simulink model "Three_blade_H_VAWT_Model"  (R2018b)
settings: Solver=FixedStepAuto  StartTime=0.0  StopTime=10  FixedStep=0.01  RelTol=1e-3
values from neighbouring files (symbols this model uses):
  A0 = 0    [Three_blade_H_VAWT_init.m]    (also in Three_blade_H_VAWT_pre_post.m)
  a1 = 0.01    [Three_blade_H_VAWT_init.m]    (also in Three_blade_H_VAWT_pre_post.m)
  a11 = 0.8    [Three_blade_H_VAWT_init.m]    (also in Three_blade_H_VAWT_pre_post.m)
  a12 = 0.2    [Three_blade_H_VAWT_init.m]    (also in Three_blade_H_VAWT_pre_post.m)
  a2 = 0.08    [Three_blade_H_VAWT_init.m]    (also in Three_blade_H_VAWT_pre_post.m)
  a21 = 0.5    [Three_blade_H_VAWT_init.m]    (also in Three_blade_H_VAWT_pre_post.m)
  a22 = 0.5    [Three_blade_H_VAWT_init.m]    (also in Three_blade_H_VAWT_pre_post.m)
  A_wind = 10    [Three_blade_H_VAWT_init.m]    (also in Three_blade_H_VAWT_pre_post.m)
  ACD1 = 12    [Three_blade_H_VAWT_init.m]    (also in Three_blade_H_VAWT_pre_post.m)
  ACL1 = 15    [Three_blade_H_VAWT_init.m]    (also in Three_blade_H_VAWT_pre_post.m)
  AR = Blade_Length/Chord    (= 10)    [Three_blade_H_VAWT_init.m]    (also in Three_blade_H_VAWT_pre_post.m = 40)
  blade1_pitch = 0    [Three_blade_H_VAWT_pre_post.m]
  blade1_radius = 20    [Three_blade_H_VAWT_pre_post.m]
  blade2_pitch = 0    [Three_blade_H_VAWT_pre_post.m]
  blade2_radius = 20    [Three_blade_H_VAWT_pre_post.m]
  blade3_pitch = 0    [Three_blade_H_VAWT_pre_post.m]
  blade3_radius = 20    [Three_blade_H_VAWT_pre_post.m]
  Blade_Length = 40    [Three_blade_H_VAWT_init.m]    (also in Three_blade_H_VAWT_pre_post.m)
  C_l_NACA0012_spline = spline(angles, C_l_NACA0012, [0:1:360])    [Three_blade_H_VAWT_init.m]    (also in Three_blade_H_VAWT_pre_post.m)
  CD0 = 0.005    [Three_blade_H_VAWT_init.m]    (also in Three_blade_H_VAWT_pre_post.m)
  CD1_max = 0.017    [Three_blade_H_VAWT_init.m]    (also in Three_blade_H_VAWT_pre_post.m)
  CD2_max = 1.8    [Three_blade_H_VAWT_init.m]    (also in Three_blade_H_VAWT_pre_post.m)
  CL1_max = 1.4    [Three_blade_H_VAWT_init.m]    (also in Three_blade_H_VAWT_pre_post.m)
  CL2_max = 1.2    [Three_blade_H_VAWT_init.m]    (also in Three_blade_H_VAWT_pre_post.m)
  D = 10^6    (= 1000000)    [Three_blade_H_VAWT_init.m]    (also in Three_blade_H_VAWT_pre_post.m)
  eta_g = 0.9    [Three_blade_H_VAWT_init.m]    (also in Three_blade_H_VAWT_pre_post.m)
  h1 = 1    [Three_blade_H_VAWT_init.m]    (also in Three_blade_H_VAWT_pre_post.m)
  h2 = 1    [Three_blade_H_VAWT_init.m]    (also in Three_blade_H_VAWT_pre_post.m)
  Jg = 15.8    [Three_blade_H_VAWT_init.m]    (also in Three_blade_H_VAWT_pre_post.m)
  K = 6*10^7    (= 60000000)    [Three_blade_H_VAWT_init.m]    (also in Three_blade_H_VAWT_pre_post.m)
  N = 100    [Three_blade_H_VAWT_init.m]    (also in Three_blade_H_VAWT_pre_post.m)
  phi11 = 0    [Three_blade_H_VAWT_init.m]    (also in Three_blade_H_VAWT_pre_post.m)
  phi12 = pi/2    (= 1.57079632679)    [Three_blade_H_VAWT_init.m]    (also in Three_blade_H_VAWT_pre_post.m)
  phi21 = 0    [Three_blade_H_VAWT_init.m]    (also in Three_blade_H_VAWT_pre_post.m)
  phi22 = pi/2    (= 1.57079632679)    [Three_blade_H_VAWT_init.m]    (also in Three_blade_H_VAWT_pre_post.m)
  Planform_A = Blade_Length*Chord    (= 160)    [Three_blade_H_VAWT_init.m]    (also in Three_blade_H_VAWT_pre_post.m = 40)
  rho = 1.225    [Three_blade_H_VAWT_init.m]    (also in Three_blade_H_VAWT_pre_post.m; sim_init_junior_project.m)
  S1 = 0.6/6    (= 0.1)    [Three_blade_H_VAWT_init.m]    (also in Three_blade_H_VAWT_pre_post.m)
  v_gustmax = v_wind    (= 5)    [Three_blade_H_VAWT_init.m]    (also in Three_blade_H_VAWT_pre_post.m)
  v_wind = 5    [Three_blade_H_VAWT_init.m]    (also in Three_blade_H_VAWT_pre_post.m)
  w_gust = (2*pi)/(30)    (= 0.209439510239)    [Three_blade_H_VAWT_init.m]    (also in Three_blade_H_VAWT_pre_post.m)
  w_wind = (2*pi)*5    (= 31.4159265359)    [Three_blade_H_VAWT_init.m]    (also in Three_blade_H_VAWT_pre_post.m)
  wind_vector_i = [50,0,0]    [Three_blade_H_VAWT_pre_post.m]
undefined symbols (not defined in the file or in its folder): Bg, C_Tg, C_Tr, c_wg, c_wr, Cg, Cr, J_g, Kg, Kr, L, magnitude, R2, Re, tau_e
libraries: vrlib x6, dspmathops x6
(part 1 of 2)
settings Model: Creator=Ryan  LastModifiedBy=Ryan
settings DataIOCC: InspectSignalLogs=on
settings SFSimCC: SimUseLocalCustomCode=off
settings RTWCC: RTWUseLocalCustomCode=off
settings CodeAppCC: StateflowObjectComments=on

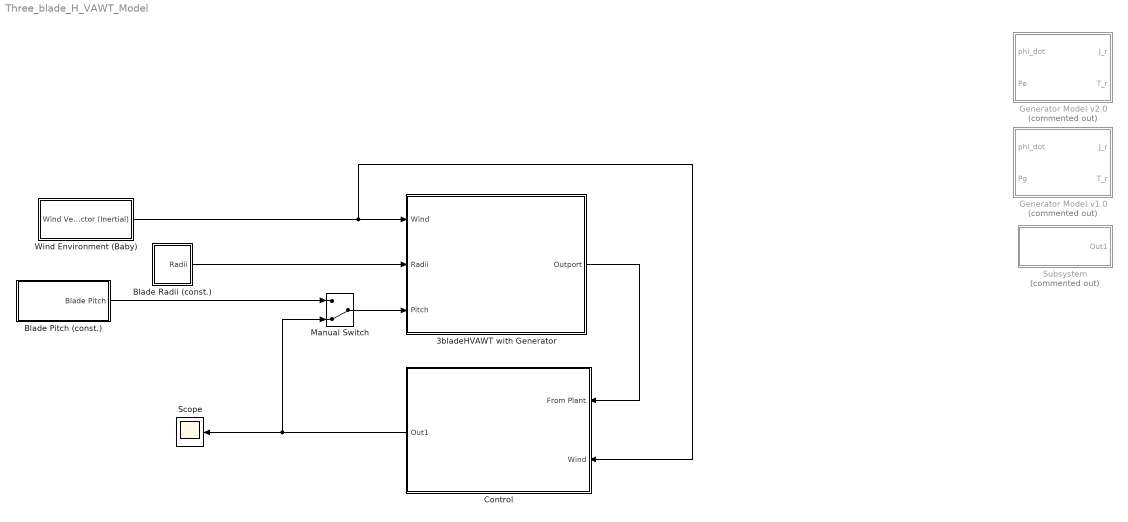
== system Three_blade_H_VAWT_Model ==
  3bladeHVAWT with Generator : Subsystem
  Blade Pitch (const.) : Subsystem
  Blade Radii (const.) : Subsystem
  Control : Subsystem
  Generator Model v1.0 : Subsystem  Commented=on
  Generator Model v2.0 : Subsystem  Commented=on
  Manual Switch : ManualSwitch  CurrentSetting=0
  Scope : Scope
  Subsystem : Subsystem  Commented=on
  Wind Environment (Baby) : Subsystem
  wires:
  3bladeHVAWT with Generator/1(Outport) -> Control/1(From Plant)
  Blade Radii (const.)/1(Radii) -> 3bladeHVAWT with Generator/2(Radii)
  Wind Environment (Baby)/1(Wind Vector (Inertial)) -> Control/2(Wind), 3bladeHVAWT with Generator/1(Wind)
  Control/1(Out1) -> Manual Switch/2, Scope/1
  Blade Pitch (const.)/1(Blade Pitch) -> Manual Switch/1
  Manual Switch/1 -> 3bladeHVAWT with Generator/3(Pitch)

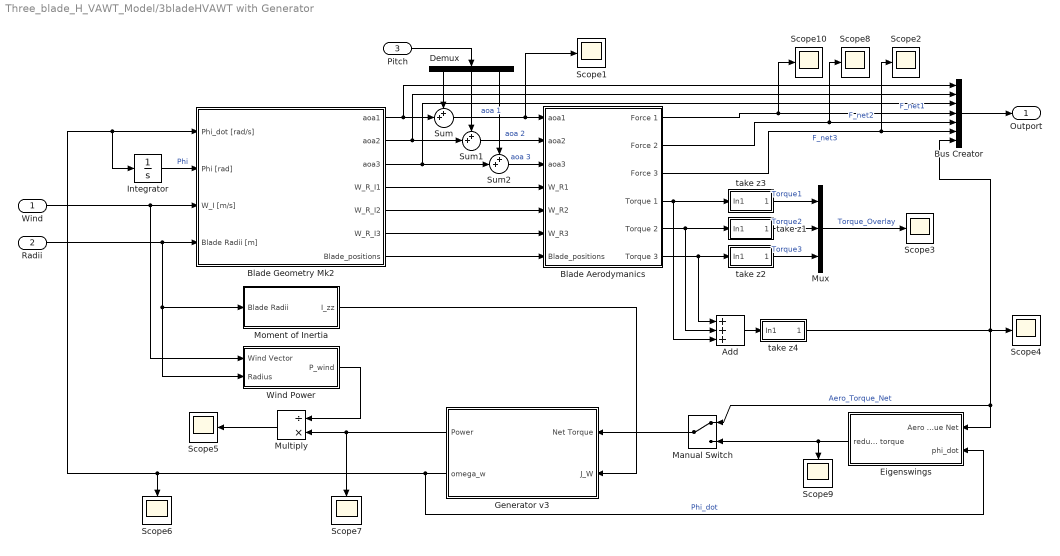
== system Three_blade_H_VAWT_Model/3bladeHVAWT with Generator ==
  Wind : Inport
  Radii : Inport  Port=2
  Pitch : Inport  Port=3
  Add : Sum  Inputs=3
  Blade Aerodymanics : Subsystem
  Blade Geometry Mk2 : Subsystem
  Bus Creator : BusCreator  Inputs=7
  Demux : Demux  Outputs=3
  Eigenswings : Subsystem
  Generator v3 : Subsystem
  Integrator : Integrator
  Manual Switch : ManualSwitch
  Moment of Inertia : Subsystem
  Multiply : Product  Inputs=/*
  Mux : Mux  Inputs=3
  Scope{1..10} (10 alike) : Scope
  Sum : Sum  Inputs=++|
  Sum1 : Sum  Inputs=++|
  Sum2 : Sum  Inputs=++|
  Wind Power : Subsystem
  take z1 : Subsystem
  take z2 : Subsystem
  take z3 : Subsystem
  take z4 : Subsystem
  Outport : Outport
  wires:
  take z4/1(Out1) -> Bus Creator/7, Eigenswings/1(Aero Torque Net), Manual Switch/1, Scope4/1  "Aero_Torque_Net"
  Blade Geometry Mk2/2(aoa2) -> Sum1/2, Bus Creator/2
  Blade Geometry Mk2/3(aoa3) -> Sum2/2, Bus Creator/3
  Radii/1 -> Blade Geometry Mk2/4(Blade Radii [m]), Moment of Inertia/1(Blade Radii), Wind Power/2(Radius)
  Pitch/1 -> Demux/1
  take z2/1(Out1) -> Mux/3  "Torque3"
  take z3/1(Out1) -> Mux/1  "Torque1"
  Wind Power/1(P_wind) -> Multiply/1
  Add/1 -> take z4/1(In1)
  Blade Aerodymanics/6(Torque 3) -> Add/1, take z2/1(In1)
  Integrator/1 -> Blade Geometry Mk2/2(Phi [rad])  "Phi"
  Blade Aerodymanics/4(Torque 1) -> Add/3, take z3/1(In1)
  take z1/1(Out1) -> Mux/2  "Torque2"
  Generator v3/1(Power) -> Multiply/2, Scope7/1
  Blade Geometry Mk2/1(aoa1) -> Sum/2, Bus Creator/1
  Wind/1 -> Wind Power/1(Wind Vector), Blade Geometry Mk2/3(W_I [m/s])
  Blade Geometry Mk2/4(W_R_I1) -> Blade Aerodymanics/4(W_R1)
  Blade Geometry Mk2/7(Blade_positions) -> Blade Aerodymanics/7(Blade_positions)
  Eigenswings/1(reduced torque) -> Manual Switch/2, Scope9/1
  Blade Aerodymanics/2(Force 2) -> Bus Creator/5, Scope8/1  "F_net2"
  Blade Aerodymanics/3(Force 3) -> Bus Creator/6, Scope2/1  "F_net3"
  Blade Aerodymanics/5(Torque 2) -> Add/2, take z1/1(In1)
  Blade Aerodymanics/1(Force 1) -> Scope10/1, Bus Creator/4  "F_net1"
  Moment of Inertia/1(I_zz) -> Generator v3/2(J_W)
  Blade Geometry Mk2/5(W_R_I2) -> Blade Aerodymanics/5(W_R2)
  Multiply/1 -> Scope5/1
  Generator v3/2(omega_w) -> Eigenswings/2(phi_dot), Integrator/1, Blade Geometry Mk2/1(Phi_dot [rad/s]), Scope6/1  "Phi_dot"
  Manual Switch/1 -> Generator v3/1(Net Torque)
  Blade Geometry Mk2/6("W_R_I3 ") -> Blade Aerodymanics/6(W_R3)
  Mux/1 -> Scope3/1  "Torque_Overlay"
  Bus Creator/1 -> Outport/1
  Demux/1 -> Sum/1
  Sum/1 -> Scope1/1, Blade Aerodymanics/1(aoa1)  "aoa 1"
  Demux/2 -> Sum1/1
  Demux/3 -> Sum2/1
  Sum2/1 -> Blade Aerodymanics/3(aoa3)  "aoa 3"
  Sum1/1 -> Blade Aerodymanics/2(aoa2)  "aoa 2"

== system Three_blade_H_VAWT_Model/Blade Pitch (const.) ==
  Constant : Constant  Value=blade1_pitch
  Constant1 : Constant  Value=blade2_pitch
  Constant2 : Constant  Value=blade3_pitch
  Mux : Mux  Inputs=3
  Blade Pitch : Outport
  wires:
  Mux/1 -> Blade Pitch/1
  Constant1/1 -> Mux/2
  Constant2/1 -> Mux/3
  Constant/1 -> Mux/1

== system Three_blade_H_VAWT_Model/Blade Radii (const.) ==
  Constant : Constant  Value=blade1_radius
  Constant1 : Constant  Value=blade2_radius
  Constant2 : Constant  Value=blade3_radius
  Mux : Mux  Inputs=3
  Radii : Outport
  wires:
  Constant/1 -> Mux/1
  Constant2/1 -> Mux/3
  Constant1/1 -> Mux/2
  Mux/1 -> Radii/1

== system Three_blade_H_VAWT_Model/Control ==
  From Plant : Inport
  Wind : Inport  Port=2
  Constant : Constant  Value=0
  Pitch Control (aoa feedback) Gain Scheduled1 : Subsystem  Commented=on
  Pitch Control (aoa feedback)1 : Subsystem  Commented=on
  Pitch Control (aoa sqrd feedback) : Subsystem  Commented=on
  Terminator : Terminator
  Terminator1 : Terminator
  Out1 : Outport
  wires:
  From Plant/1 -> Terminator1/1
  Constant/1 -> Out1/1
  Wind/1 -> Terminator/1

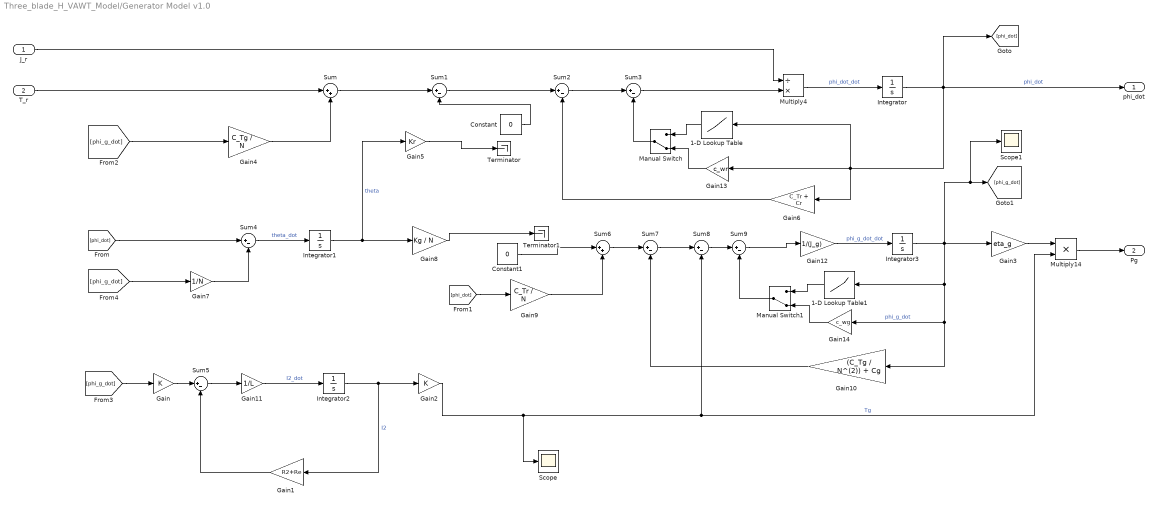
== system Three_blade_H_VAWT_Model/Generator Model v1.0 ==
  J_r : Inport
  T_r : Inport  Port=2
  1-D Lookup Table : Lookup_n-D  NumberOfTableDimensions=1  BreakpointsForDimension1=[-5:5]  Table=tanh([-5:5])  InternalRulePriority=Speed  RndMeth=Simplest  InputSameDT=on
  1-D Lookup Table1 : Lookup_n-D  NumberOfTableDimensions=1  BreakpointsForDimension1=[-5:5]  Table=tanh([-5:5])  InternalRulePriority=Speed  RndMeth=Simplest  InputSameDT=on
  Constant : Constant  Value=0
  Constant1 : Constant  Value=0
  Gain : Gain  Gain=K
  Gain1 : Gain  Gain=R2+Re
  Gain10 : Gain  Gain=(C_Tg / N^(2)) + Cg
  Gain11 : Gain  Gain=1/L
  Gain12 : Gain  Gain=1/(J_g)
  Gain13 : Gain  Gain=c_wr
  Gain14 : Gain  Gain=c_wg
  Gain2 : Gain  Gain=K
  Gain3 : Gain  Gain=eta_g
  Gain4 : Gain  Gain=C_Tg / N
  Gain5 : Gain  Gain=Kr
  Gain6 : Gain  Gain=C_Tr + Cr
  Gain7 : Gain  Gain=1/N
  Gain8 : Gain  Gain=Kg / N
  Gain9 : Gain  Gain=C_Tr / N
  Integrator : Integrator  InitialCondition=.1
  Integrator1 : Integrator
  Integrator2 : Integrator
  Integrator3 : Integrator  InitialCondition=6
  Manual Switch : ManualSwitch  CurrentSetting=0
  Manual Switch1 : ManualSwitch  CurrentSetting=0
  Multiply14 : Product
  Multiply4 : Product  Inputs=/*
  Scope : Scope
  Scope1 : Scope
  Sum : Sum  Inputs=|++
  Sum{1..5,7..9} (8 alike) : Sum  Inputs=|+-
  Sum6 : Sum  Inputs=|++
  Terminator : Terminator
  Terminator1 : Terminator
  phi_dot : Outport
  "Pg " : Outport  Port=2
  wires:
  T_r/1 -> Sum/1
  Gain4/1 -> Sum/2
  Sum/1 -> Sum1/1
  Sum1/1 -> Sum2/1
  J_r/1 -> Multiply4/1
  Multiply4/1 -> Integrator/1  "phi_dot_dot"
  Integrator/1 -> [phi_dot], Gain13/1, 1-D Lookup Table/1, Gain6/1, phi_dot/1  "phi_dot"
  [phi_dot] -> Sum4/1
  Sum4/1 -> Integrator1/1  "theta_dot"
  Integrator1/1 -> Gain8/1, Gain5/1  "theta"
  Sum6/1 -> Sum7/1
  Integrator3/1 -> Gain14/1, Gain10/1, 1-D Lookup Table1/1, Gain3/1, Scope1/1, [phi_g_dot]  "phi_g_dot"
  Sum7/1 -> Sum8/1
  [phi_g_dot] -> Gain/1
  Gain/1 -> Sum5/1
  Gain1/1 -> Sum5/2
  Integrator2/1 -> Gain2/1, Gain1/1  "I2"
  Sum5/1 -> Gain11/1
  Gain11/1 -> Integrator2/1  "I2_dot"
  Gain2/1 -> Scope/1, Sum8/2, Multiply14/2  "Tg"
  Gain12/1 -> Integrator3/1  "phi_g_dot_dot"
  Gain3/1 -> Multiply14/1
  Multiply14/1 -> "Pg "/1
  [phi_g_dot] -> Gain4/1
  Gain6/1 -> Sum2/2
  [phi_g_dot] -> Gain7/1
  Gain7/1 -> Sum4/2
  [phi_dot] -> Gain9/1
  Gain9/1 -> Sum6/2
  Gain10/1 -> Sum7/2
  Sum2/1 -> Sum3/1
  Sum3/1 -> Multiply4/2
  Sum8/1 -> Sum9/1
  Sum9/1 -> Gain12/1
  Manual Switch/1 -> Sum3/2
  1-D Lookup Table/1 -> Manual Switch/1
  Gain13/1 -> Manual Switch/2
  Manual Switch1/1 -> Sum9/2
  1-D Lookup Table1/1 -> Manual Switch1/1
  Gain14/1 -> Manual Switch1/2
  Gain5/1 -> Terminator/1
  Gain8/1 -> Terminator1/1
  Constant/1 -> Sum1/2
  Constant1/1 -> Sum6/1

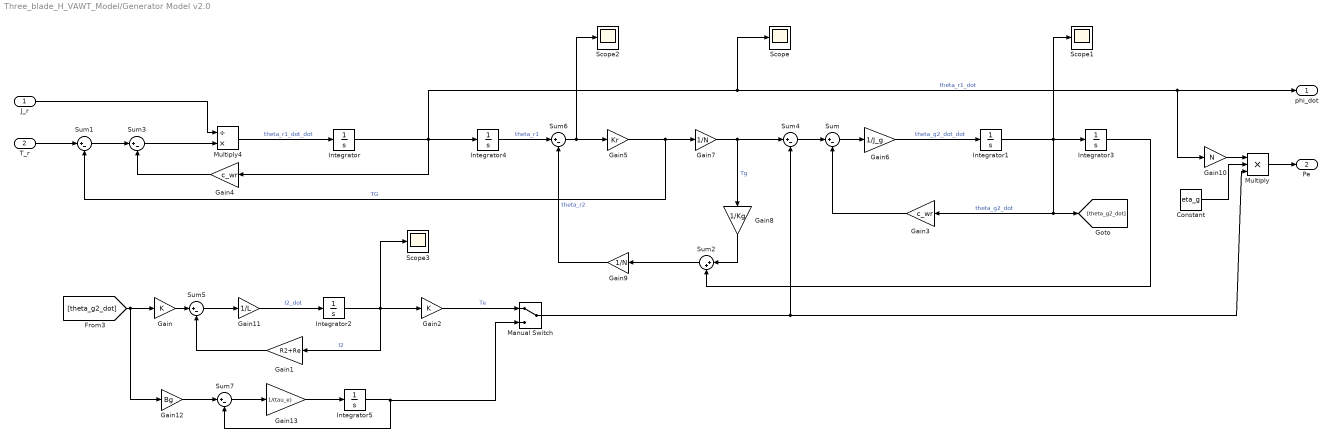
== system Three_blade_H_VAWT_Model/Generator Model v2.0 ==
  J_r : Inport
  T_r : Inport  Port=2
  Constant : Constant  Value=eta_g
  Gain : Gain  Gain=K
  Gain1 : Gain  Gain=R2+Re
  Gain10 : Gain  Gain=N
  Gain11 : Gain  Gain=1/L
  Gain12 : Gain  Gain=Bg
  Gain13 : Gain  Gain=1/(tau_e)
  Gain2 : Gain  Gain=K
  Gain3 : Gain  Gain=c_wr
  Gain4 : Gain  Gain=c_wr
  Gain5 : Gain  Gain=Kr
  Gain6 : Gain  Gain=1/J_g
  Gain7 : Gain  Gain=1/N
  Gain8 : Gain  Gain=1/Kg
  Gain9 : Gain  Gain=1/N
  Integrator{,1..5} (6 alike) : Integrator
  Manual Switch : ManualSwitch
  Multiply : Product  Inputs=3
  Multiply4 : Product  Inputs=/*
  Scope{,1..3} (4 alike) : Scope
  Sum{,1,3..7} (7 alike) : Sum  Inputs=|+-
  Sum2 : Sum  Inputs=|++
  phi_dot : Outport
  Pe : Outport  Port=2
  wires:
  J_r/1 -> Multiply4/1
  Multiply4/1 -> Integrator/1  "theta_r1_dot_dot"
  Integrator/1 -> Integrator4/1, Gain4/1, Scope/1, phi_dot/1, Gain10/1  "theta_r1_dot"
  [theta_g2_dot] -> Gain12/1, Gain/1
  Gain/1 -> Sum5/1
  Gain1/1 -> Sum5/2
  Integrator2/1 -> Scope3/1, Gain2/1, Gain1/1  "I2"
  Sum5/1 -> Gain11/1
  Gain11/1 -> Integrator2/1  "I2_dot"
  Sum3/1 -> Multiply4/2
  Integrator4/1 -> Sum6/1  "theta_r1"
  T_r/1 -> Sum1/1
  Sum1/1 -> Sum3/1
  Gain4/1 -> Sum3/2
  Sum6/1 -> Scope2/1, Gain5/1
  Gain5/1 -> Gain7/1, Sum1/2  "TG"
  Gain7/1 -> Gain8/1, Sum4/1  "Tg"
  Sum4/1 -> Sum/1
  Gain3/1 -> Sum/2
  Sum/1 -> Gain6/1
  Gain6/1 -> Integrator1/1  "theta_g2_dot_dot"
  Integrator1/1 -> Scope1/1, Gain3/1, [theta_g2_dot], Integrator3/1  "theta_g2_dot"
  Integrator3/1 -> Sum2/2
  Gain8/1 -> Sum2/1
  Sum2/1 -> Gain9/1
  Gain9/1 -> Sum6/2  "theta_r2"
  Gain10/1 -> Multiply/1
  Multiply/1 -> Pe/1
  Constant/1 -> Multiply/2
  Gain2/1 -> Manual Switch/1  "Te"
  Manual Switch/1 -> Sum4/2, Multiply/3
  Gain12/1 -> Sum7/1
  Integrator5/1 -> Manual Switch/2, Sum7/2
  Gain13/1 -> Integrator5/1
  Sum7/1 -> Gain13/1

== system Three_blade_H_VAWT_Model/Subsystem ==
  Clock : Clock
  Constant : Constant
  Constant1 : Constant  Value=2*v_gustmax
  Constant2 : Constant
  Exp : Math  SaturateOnIntegerOverflow=on
  Gain : Gain  Gain=w_wind
  Gain1 : Gain  Gain=w_gust
  Gain2 : Gain  Gain=-4
  Gain3 : Gain  Gain=A_wind
  Gain4 : Gain  Gain=v_wind
  Multiply : Product  Inputs=*/
  Scope : Scope
  Sin : Trigonometry
  Sin1 : Trigonometry
  Sum : Sum
  Sum1 : Sum  Inputs=|++
  Sum2 : Sum  Inputs=|+-
  Sum3 : Sum  Inputs=|+-
  Out1 : Outport
  wires:
  Clock/1 -> Gain1/1, Gain/1
  Gain/1 -> Sin/1
  Gain1/1 -> Sin1/1
  Sin1/1 -> Sum2/1
  Constant/1 -> Sum3/2, Sum2/2
  Sum2/1 -> Gain2/1
  Constant1/1 -> Multiply/1
  Sum1/1 -> Scope/1, Out1/1
  Constant2/1 -> Sum/1
  Sin/1 -> Gain3/1
  Gain3/1 -> Sum/2
  Gain4/1 -> Sum1/1
  Sum/1 -> Gain4/1
  Gain2/1 -> Exp/1
  Exp/1 -> Sum3/1
  Sum3/1 -> Multiply/2
  Multiply/1 -> Sum1/2

== system Three_blade_H_VAWT_Model/Wind Environment (Baby) ==
  Constant : Constant  Value=wind_vector_i
  Wind Vector (Inertial) : Outport
  wires:
  Constant/1 -> Wind Vector (Inertial)/1

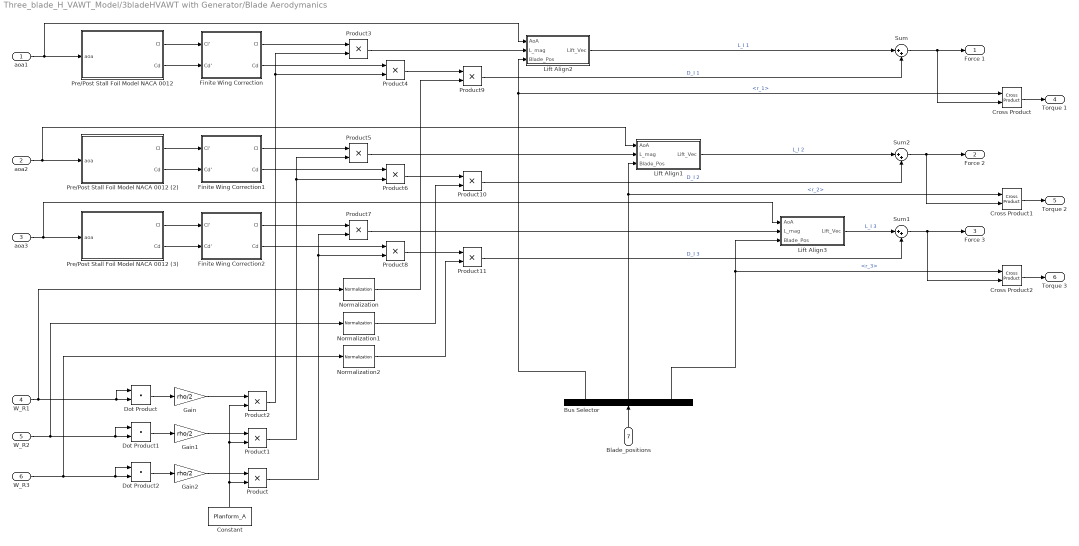
== system Three_blade_H_VAWT_Model/3bladeHVAWT with Generator/Blade Aerodymanics ==
  aoa1 : Inport
  aoa2 : Inport  Port=2
  aoa3 : Inport  Port=3
  W_R1 : Inport  Port=4
  W_R2 : Inport  Port=5
  W_R3 : Inport  Port=6
  Blade_positions : Inport  Port=7
  Bus Selector : BusSelector  OutputSignals=r_1,r_2,r_3
  Constant : Constant  Value=Planform_A
  Cross Product : vrlib/Utilities/Cross Product
      settings: SourceProductBaseCode=VR
  Cross Product1 : vrlib/Utilities/Cross Product
      settings: SourceProductBaseCode=VR
  Cross Product2 : vrlib/Utilities/Cross Product
      settings: SourceProductBaseCode=VR
  Dot Product : DotProduct  InputSameDT=on  OutDataTypeStr=Inherit: Inherit via internal rule
  Dot Product1 : DotProduct  InputSameDT=on  OutDataTypeStr=Inherit: Inherit via internal rule
  Dot Product2 : DotProduct  InputSameDT=on  OutDataTypeStr=Inherit: Inherit via internal rule
  Finite Wing Correction : Subsystem
  Finite Wing Correction1 : Subsystem
  Finite Wing Correction2 : Subsystem
  Gain : Gain  Gain=rho/2
  Gain1 : Gain  Gain=rho/2
  Gain2 : Gain  Gain=rho/2
  Lift Align1 : Subsystem
  Lift Align2 : Subsystem
  Lift Align3 : Subsystem
  Normalization : dspmathops/Normalization  NormType=2-norm  Bias=1e-10  NormOver=Each column  Dimension=1  roundingMode=Floor  overflowMode=off  accumDataTypeStr=Inherit: Same as product output  accumLastDataTypeStr=Inherit: Same as product output  outputDataTypeStr=Inherit: Same as product output  outputMin=[]  outputMax=[]  outputLastDataTypeStr=Inherit: Same as product output
      settings: SourceProductName=DSP System Toolbox
  Normalization1 : dspmathops/Normalization  NormType=2-norm  Bias=1e-10  NormOver=Each column  Dimension=1  roundingMode=Floor  overflowMode=off  accumDataTypeStr=Inherit: Same as product output  accumLastDataTypeStr=Inherit: Same as product output  outputDataTypeStr=Inherit: Same as product output  outputMin=[]  outputMax=[]  outputLastDataTypeStr=Inherit: Same as product output
      settings: SourceProductName=DSP System Toolbox
  Normalization2 : dspmathops/Normalization  NormType=2-norm  Bias=1e-10  NormOver=Each column  Dimension=1  roundingMode=Floor  overflowMode=off  accumDataTypeStr=Inherit: Same as product output  accumLastDataTypeStr=Inherit: Same as product output  outputDataTypeStr=Inherit: Same as product output  outputMin=[]  outputMax=[]  outputLastDataTypeStr=Inherit: Same as product output
      settings: SourceProductName=DSP System Toolbox
  Pre/Post Stall Foil Model NACA 0012 : Subsystem
  Pre/Post Stall Foil Model NACA 0012 (2) : Subsystem
  Pre/Post Stall Foil Model NACA 0012 (3) : Subsystem
  Product{,1..11} (12 alike) : Product
  Sum : Sum  Inputs=|++
  Sum1 : Sum  Inputs=|++
  Sum2 : Sum  Inputs=|++
  Force 1 : Outport
  Force 2 : Outport  Port=2
  Force 3 : Outport  Port=3
  Torque 1 : Outport  Port=4
  Torque 2 : Outport  Port=5
  Torque 3 : Outport  Port=6
  wires:
  aoa1/1 -> Lift Align2/1(AoA), Pre/Post Stall Foil Model NACA 0012/1(aoa)
  aoa2/1 -> Lift Align1/1(AoA), Pre/Post Stall Foil Model NACA 0012 (2)/1(aoa)
  aoa3/1 -> Lift Align3/1(AoA), Pre/Post Stall Foil Model NACA 0012 (3)/1(aoa)
  Pre/Post Stall Foil Model NACA 0012/1(Cl) -> Finite Wing Correction/1(Cl')
  Pre/Post Stall Foil Model NACA 0012/2(Cd) -> Finite Wing Correction/2(Cd')
  Pre/Post Stall Foil Model NACA 0012 (3)/2(Cd) -> Finite Wing Correction2/2(Cd')
  Pre/Post Stall Foil Model NACA 0012 (3)/1(Cl) -> Finite Wing Correction2/1(Cl')
  Pre/Post Stall Foil Model NACA 0012 (2)/2(Cd) -> Finite Wing Correction1/2(Cd')
  Pre/Post Stall Foil Model NACA 0012 (2)/1(Cl) -> Finite Wing Correction1/1(Cl')
  W_R1/1 -> Dot Product/1, Dot Product/2, Normalization/1
  W_R2/1 -> Dot Product1/1, Dot Product1/2, Normalization1/1
  W_R3/1 -> Normalization2/1, Dot Product2/1, Dot Product2/2
  Dot Product/1 -> Gain/1
  Dot Product2/1 -> Gain2/1
  Dot Product1/1 -> Gain1/1
  Gain/1 -> Product2/1
  Gain1/1 -> Product1/1
  Gain2/1 -> Product/1
  Constant/1 -> Product/2, Product2/2, Product1/2
  Finite Wing Correction/2(Cd) -> Product4/1
  Finite Wing Correction/1(Cl) -> Product3/1
  Finite Wing Correction1/2(Cd) -> Product6/1
  Finite Wing Correction1/1(Cl) -> Product5/1
  Finite Wing Correction2/2(Cd) -> Product8/1
  Finite Wing Correction2/1(Cl) -> Product7/1
  Product2/1 -> Product4/2, Product3/2
  Product1/1 -> Product6/2, Product5/2
  Product/1 -> Product8/2, Product7/2
  Product4/1 -> Product9/1
  Normalization/1 -> Product9/2
  Product6/1 -> Product10/1
  Product8/1 -> Product11/1
  Normalization1/1 -> Product10/2
  Normalization2/1 -> Product11/2
  Product9/1 -> Sum/2  "D_I 1"
  Product10/1 -> Sum2/2  "D_I 2"
  Product11/1 -> Sum1/2  "D_I 3"
  Sum/1 -> Cross Product/2, Force 1/1
  Sum2/1 -> Cross Product1/2, Force 2/1
  Sum1/1 -> Cross Product2/2, Force 3/1
  Blade_positions/1 -> Bus Selector/1
  Product7/1 -> Lift Align3/2(L_mag)
  Bus Selector/1 -> Cross Product/1, Lift Align2/3(Blade_Pos)  "<r_1>"
  Product5/1 -> Lift Align1/2(L_mag)
  Bus Selector/2 -> Cross Product1/1, Lift Align1/3(Blade_Pos)  "<r_2>"
  Product3/1 -> Lift Align2/2(L_mag)
  Bus Selector/3 -> Cross Product2/1, Lift Align3/3(Blade_Pos)  "<r_3>"
  Lift Align3/1(Lift_Vec) -> Sum1/1  "L_I 3"
  Lift Align1/1(Lift_Vec) -> Sum2/1  "L_I 2"
  Lift Align2/1(Lift_Vec) -> Sum/1  "L_I 1"
  Cross Product/1 -> Torque 1/1
  Cross Product1/1 -> Torque 2/1
  Cross Product2/1 -> Torque 3/1

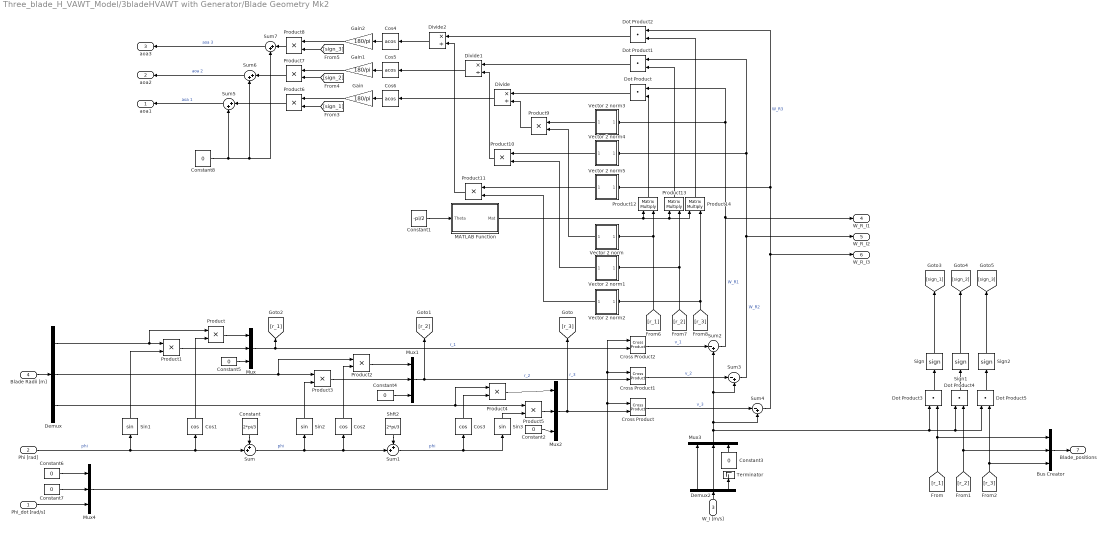
== system Three_blade_H_VAWT_Model/3bladeHVAWT with Generator/Blade Geometry Mk2 ==
  Phi_dot [rad/s] : Inport
  Phi [rad] : Inport  Port=2
  W_I [m/s] : Inport  Port=3
  Blade Radii [m] : Inport  Port=4
  Bus Creator : BusCreator  Inputs=3
  Constant : Constant  Value=2*pi/3
  Constant1 : Constant  Value=-pi/2
  Constant{2..8} (7 alike) : Constant  Value=0
  Cos1 : Trigonometry  Operator=cos
  Cos2 : Trigonometry  Operator=cos
  Cos3 : Trigonometry  Operator=cos
  Cos4 : Trigonometry  Operator=acos
  Cos5 : Trigonometry  Operator=acos
  Cos6 : Trigonometry  Operator=acos
  Cross Product : vrlib/Utilities/Cross Product
      settings: SourceProductBaseCode=VR
  Cross Product1 : vrlib/Utilities/Cross Product
      settings: SourceProductBaseCode=VR
  Cross Product2 : vrlib/Utilities/Cross Product
      settings: SourceProductBaseCode=VR
  Demux : Demux  Outputs=3
  Demux2 : Demux  Outputs=3
  Divide : Product  Inputs=*/
  Divide1 : Product  Inputs=*/
  Divide2 : Product  Inputs=*/
  Dot Product{,1..5} (6 alike) : DotProduct  InputSameDT=on  OutDataTypeStr=Inherit: Inherit via internal rule
  Gain : Gain  Gain=180/pi
  Gain1 : Gain  Gain=180/pi
  Gain2 : Gain  Gain=180/pi
  MATLAB Function : MATLAB Function  TreatAsAtomicUnit=on
  Mux{,1..4} (5 alike) : Mux  Inputs=3
  Product{,1..11} (12 alike) : Product
  Product12 : Product  Multiplication=Matrix(*)
  Product13 : Product  Multiplication=Matrix(*)
  Product14 : Product  Multiplication=Matrix(*)
  Shft2 : Constant  Value=2*pi/3
  Sign : Signum
  Sign1 : Signum
  Sign2 : Signum
  Sin1 : Trigonometry
  Sin2 : Trigonometry
  Sin3 : Trigonometry
  Sum : Sum  Inputs=++|
  Sum1 : Sum  Inputs=++|
  Sum2 : Sum  Inputs=|-+
  Sum3 : Sum  Inputs=|-+
  Sum4 : Sum  Inputs=|-+
  Sum5 : Sum  Inputs=|++
  Sum6 : Sum  Inputs=|++
  Sum7 : Sum  Inputs=|++
  Terminator : Terminator
  Vector 2 norm : Subsystem
  Vector 2 norm1 : Subsystem
  Vector 2 norm2 : Subsystem
  Vector 2 norm3 : Subsystem
  Vector 2 norm4 : Subsystem
  Vector 2 norm5 : Subsystem
  aoa1 : Outport
  aoa2 : Outport  Port=2
  aoa3 : Outport  Port=3
  W_R_I1 : Outport  Port=4
  W_R_I2 : Outport  Port=5
  "W_R_I3 " : Outport  Port=6
  Blade_positions : Outport  Port=7
  wires:
  Mux4/1 -> Cross Product2/1, Cross Product1/1, Cross Product/1
  Dot Product/1 -> Divide/1
  Sum2/1 -> W_R_I1/1, Dot Product/1, Vector 2 norm3/1(In1)  "W_R1"
  Mux1/1 -> Cross Product1/2, [r_2]  "r_2"
  Product/1 -> Mux/1
  Sin1/1 -> Product1/2
  Product1/1 -> Mux/2
  Sum/1 -> Sum1/2, Cos2/1, Sin2/1  "phi"
  Cos1/1 -> Product/2
  Sum1/1 -> Sin3/1, Cos3/1  "phi"
  Sin2/1 -> Product3/2
  Product3/1 -> Mux1/2
  Cos2/1 -> Product2/2
  Product2/1 -> Mux1/1
  Demux/3 -> Product4/1, Product5/1
  Cross Product2/1 -> Sum2/1  "v_1"
  Sum4/1 -> Dot Product2/1, Vector 2 norm5/1(In1), "W_R_I3 "/1  "W_R3"
  Product4/1 -> Mux2/1
  Sin3/1 -> Product5/2
  Product5/1 -> Mux2/2
  Cos3/1 -> Product4/2
  Shft2/1 -> Sum1/1
  Demux/1 -> Product/1, Product1/1
  Demux/2 -> Product2/1, Product3/1
  Vector 2 norm5/1(Out1) -> Product11/1
  Sum7/1 -> aoa3/1  "aoa 3"
  Divide/1 -> Cos6/1
  Dot Product2/1 -> Divide2/1
  Phi [rad]/1 -> Sum/2, Cos1/1, Sin1/1  "phi"
  Constant/1 -> Sum/1
  Cos4/1 -> Gain2/1
  Vector 2 norm2/1(Out1) -> Product11/2
  Product11/1 -> Divide2/2
  Divide1/1 -> Cos5/1
  Product10/1 -> Divide1/2
  Sum3/1 -> Dot Product1/1, Vector 2 norm4/1(In1), W_R_I2/1  "W_R2"
  Cross Product1/1 -> Sum3/1  "v_2"
  Mux2/1 -> Cross Product/2, [r_3]  "r_3"
  Cross Product/1 -> Sum4/1  "v_3"
  Mux/1 -> [r_1], Cross Product2/2  "r_1"
  Vector 2 norm4/1(Out1) -> Product10/1
  Divide2/1 -> Cos4/1
  Product9/1 -> Divide/2
  Constant8/1 -> Sum7/2, Sum6/2, Sum5/2
  Vector 2 norm1/1(Out1) -> Product10/2
  Vector 2 norm/1(Out1) -> Product9/2
  Cos6/1 -> Gain/1
  Sum6/1 -> aoa2/1  "aoa 2"
  Cos5/1 -> Gain1/1
  Sum5/1 -> aoa1/1  "aoa 1"
  Vector 2 norm3/1(Out1) -> Product9/1
  Dot Product1/1 -> Divide1/1
  Blade Radii [m]/1 -> Demux/1
  Demux2/1 -> Mux3/1
  Demux2/2 -> Mux3/2
  Demux2/3 -> Terminator/1
  W_I [m/s]/1 -> Demux2/1
  Gain/1 -> Product6/1
  Gain1/1 -> Product7/1
  Gain2/1 -> Product8/1
  Constant2/1 -> Mux2/3
  Constant3/1 -> Mux3/3
  Constant4/1 -> Mux1/3
  Constant5/1 -> Mux/3
  Phi_dot [rad/s]/1 -> Mux4/3
  Constant6/1 -> Mux4/1
  Constant7/1 -> Mux4/2
  Product12/1 -> Dot Product/2
  [r_3] -> Product14/2, Vector 2 norm2/1(In1)
  Product13/1 -> Dot Product1/2
  Product8/1 -> Sum7/1
  Product6/1 -> Sum5/1
  Product7/1 -> Sum6/1
  [sign_1] -> Product6/2
  [sign_2] -> Product7/2
  [sign_3] -> Product8/2
  Mux3/1 -> Dot Product3/1, Dot Product4/1, Dot Product5/1, Sum2/2, Sum3/2, Sum4/2
  [r_1] -> Bus Creator/1, Dot Product3/2
  [r_2] -> Bus Creator/2, Dot Product4/2
  [r_3] -> Bus Creator/3, Dot Product5/2
  Dot Product4/1 -> Sign1/1
  Dot Product3/1 -> Sign/1
  Dot Product5/1 -> Sign2/1
  Sign/1 -> [sign_1]
  Sign1/1 -> [sign_2]
  Sign2/1 -> [sign_3]
  Bus Creator/1 -> Blade_positions/1
  [r_1] -> Product12/2, Vector 2 norm/1(In1)
  [r_2] -> Product13/2, Vector 2 norm1/1(In1)
  Product14/1 -> Dot Product2/2
  Constant1/1 -> MATLAB Function/1(Theta)
  MATLAB Function/1(Mat) -> Product12/1, Product13/1, Product14/1

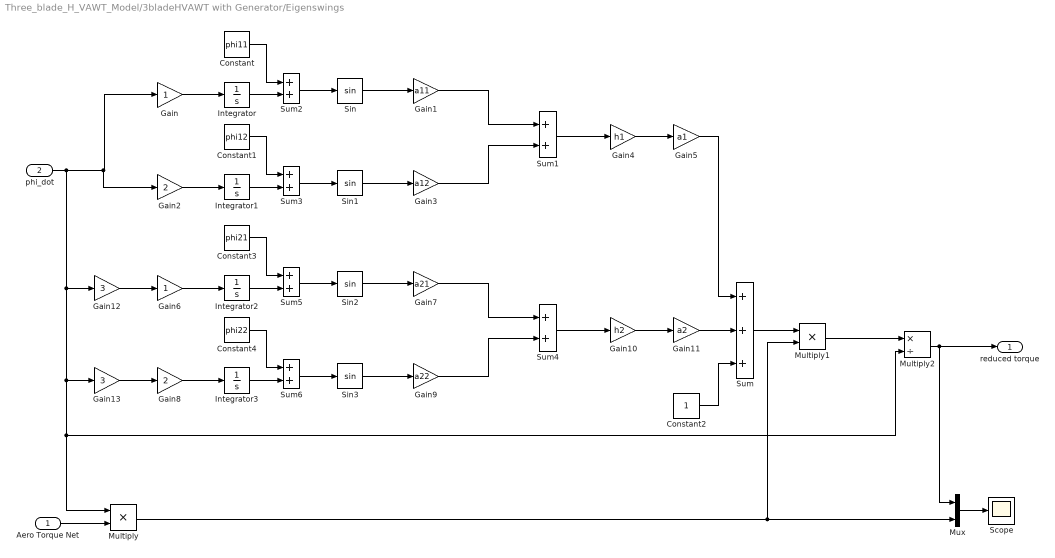
== system Three_blade_H_VAWT_Model/3bladeHVAWT with Generator/Eigenswings ==
  Aero Torque Net : Inport
  phi_dot : Inport  Port=2
  Constant : Constant  Value=phi11
  Constant1 : Constant  Value=phi12
  Constant2 : Constant
  Constant3 : Constant  Value=phi21
  Constant4 : Constant  Value=phi22
  Gain : Gain
  Gain1 : Gain  Gain=a11
  Gain10 : Gain  Gain=h2
  Gain11 : Gain  Gain=a2
  Gain12 : Gain  Gain=3
  Gain13 : Gain  Gain=3
  Gain2 : Gain  Gain=2
  Gain3 : Gain  Gain=a12
  Gain4 : Gain  Gain=h1
  Gain5 : Gain  Gain=a1
  Gain6 : Gain
  Gain7 : Gain  Gain=a21
  Gain8 : Gain  Gain=2
  Gain9 : Gain  Gain=a22
  Integrator{,1..3} (4 alike) : Integrator
  Multiply : Product
  Multiply1 : Product
  Multiply2 : Product  Inputs=*/
  Mux : Mux  Inputs=2
  Scope : Scope
  Sin{,1..3} (4 alike) : Trigonometry
  Sum : Sum  Inputs=+++
  Sum{1..6} (6 alike) : Sum
  reduced torque : Outport
  wires:
  Gain/1 -> Integrator/1
  phi_dot/1 -> Gain13/1, Multiply2/2, Multiply/1, Gain12/1, Gain2/1, Gain/1
  Integrator/1 -> Sum2/2
  Constant/1 -> Sum2/1
  Sum2/1 -> Sin/1
  Sin/1 -> Gain1/1
  Gain1/1 -> Sum1/1
  Integrator1/1 -> Sum3/2
  Gain2/1 -> Integrator1/1
  Gain3/1 -> Sum1/2
  Sum3/1 -> Sin1/1
  Sin1/1 -> Gain3/1
  Constant1/1 -> Sum3/1
  Sum1/1 -> Gain4/1
  Aero Torque Net/1 -> Multiply/2
  Sum/1 -> Multiply1/1
  Multiply/1 -> Multiply1/2, Mux/2
  Gain4/1 -> Gain5/1
  Integrator2/1 -> Sum5/2
  Gain6/1 -> Integrator2/1
  Gain7/1 -> Sum4/1
  Constant3/1 -> Sum5/1
  Gain10/1 -> Gain11/1
  Sin3/1 -> Gain9/1
  Sum5/1 -> Sin2/1
  Sin2/1 -> Gain7/1
  Constant4/1 -> Sum6/1
  Sum6/1 -> Sin3/1
  Gain9/1 -> Sum4/2
  Sum4/1 -> Gain10/1
  Gain8/1 -> Integrator3/1
  Integrator3/1 -> Sum6/2
  Gain12/1 -> Gain6/1
  Gain13/1 -> Gain8/1
  Gain11/1 -> Sum/2
  Gain5/1 -> Sum/1
  Constant2/1 -> Sum/3
  Multiply1/1 -> Multiply2/1
  Multiply2/1 -> Mux/1, reduced torque/1
  Mux/1 -> Scope/1

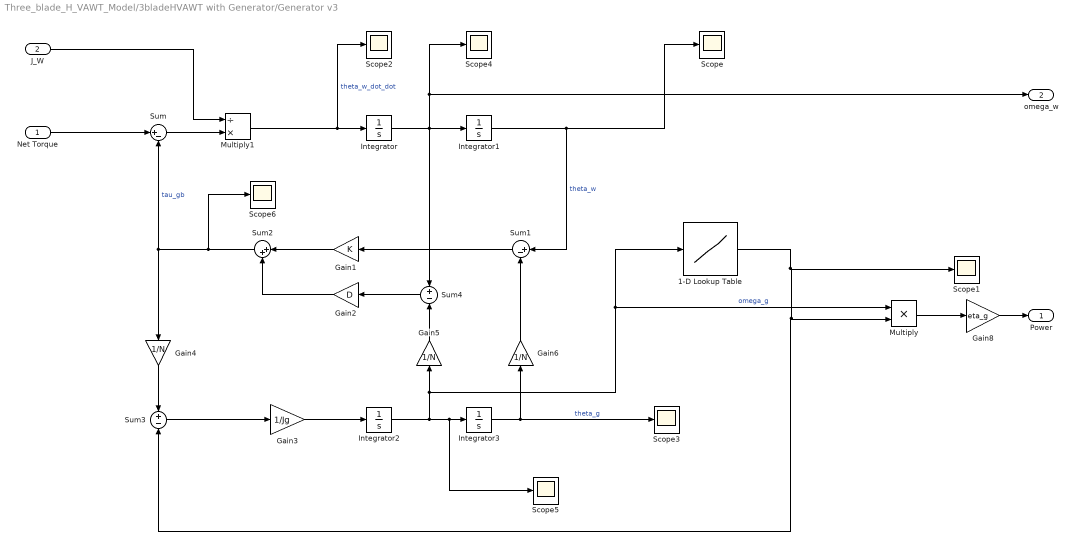
== system Three_blade_H_VAWT_Model/3bladeHVAWT with Generator/Generator v3 ==
  Net Torque : Inport
  J_W : Inport  Port=2
  1-D Lookup Table : Lookup_n-D  NumberOfTableDimensions=1  BreakpointsForDimension1=[0,104.7,107.3]  Table=[0,0,8000]  InternalRulePriority=Speed  RndMeth=Simplest  InputSameDT=on
  Gain1 : Gain  Gain=K
  Gain2 : Gain  Gain=D
  Gain3 : Gain  Gain=1/Jg
  Gain4 : Gain  Gain=1/N
  Gain5 : Gain  Gain=1/N
  Gain6 : Gain  Gain=1/N
  Gain8 : Gain  Gain=eta_g
  Integrator : Integrator  InitialCondition=106/N
  Integrator1 : Integrator
  Integrator2 : Integrator  InitialCondition=106
  Integrator3 : Integrator
  Multiply : Product
  Multiply1 : Product  Inputs=/*
  Scope{,1..6} (7 alike) : Scope
  Sum : Sum  Inputs=|+-
  Sum1 : Sum  Inputs=|+-
  Sum2 : Sum  Inputs=|++
  Sum3 : Sum  Inputs=+-
  Sum4 : Sum  Inputs=+-
  Power : Outport
  omega_w : Outport  Port=2
  wires:
  Integrator2/1 -> Scope5/1, Integrator3/1, Multiply/1, 1-D Lookup Table/1, Gain5/1  "omega_g"
  Sum4/1 -> Gain2/1
  Multiply1/1 -> Integrator/1, Scope2/1  "theta_w_dot_dot"
  Gain4/1 -> Sum3/1
  Gain6/1 -> Sum1/2
  Gain3/1 -> Integrator2/1
  Gain1/1 -> Sum2/1
  Multiply/1 -> Gain8/1
  Integrator1/1 -> Sum1/1, Scope/1  "theta_w"
  Integrator3/1 -> Gain6/1, Scope3/1  "theta_g"
  Gain2/1 -> Sum2/2
  Integrator/1 -> Sum4/1, Integrator1/1, omega_w/1, Scope4/1
  Sum2/1 -> Scope6/1, Gain4/1, Sum/2  "tau_gb"
  Net Torque/1 -> Sum/1
  Sum3/1 -> Gain3/1
  Sum1/1 -> Gain1/1
  1-D Lookup Table/1 -> Sum3/2, Multiply/2, Scope1/1
  Gain8/1 -> Power/1
  Gain5/1 -> Sum4/2
  Sum/1 -> Multiply1/2
  J_W/1 -> Multiply1/1

== system Three_blade_H_VAWT_Model/3bladeHVAWT with Generator/Moment of Inertia ==
  Blade Radii : Inport
  Add : Sum  Inputs=3
  Demux : Demux  Outputs=3
  Math Function : Math  Operator=magnitude^2  SaturateOnIntegerOverflow=on
  Math Function1 : Math  Operator=magnitude^2  SaturateOnIntegerOverflow=on
  Math Function2 : Math  Operator=magnitude^2  SaturateOnIntegerOverflow=on
  blade mass : Gain  Gain=15000
  blade mass1 : Gain  Gain=15000
  blade mass2 : Gain  Gain=15000
  I_zz : Outport
  wires:
  Blade Radii/1 -> Demux/1
  Demux/1 -> Math Function/1
  Demux/3 -> Math Function2/1
  Demux/2 -> Math Function1/1
  Math Function/1 -> blade mass/1
  Math Function1/1 -> blade mass1/1
  Math Function2/1 -> blade mass2/1
  blade mass1/1 -> Add/2
  blade mass/1 -> Add/1
  blade mass2/1 -> Add/3
  Add/1 -> I_zz/1

== system Three_blade_H_VAWT_Model/3bladeHVAWT with Generator/Wind Power ==
  Wind Vector : Inport
  Radius : Inport  Port=2
  Constant : Constant  Value=3
  Demux : Demux  Outputs=3
  Demux1 : Demux  Outputs=3
  Gain : Gain  Gain=(rho*Blade_Length)/2
  Gain1 : Gain  Gain=2
  Math Function : Math  Operator=pow  SaturateOnIntegerOverflow=on
  Multiply : Product
  Sqrt : Sqrt  SaturateOnIntegerOverflow=on
  Square : Math  Operator=square  SaturateOnIntegerOverflow=on
  Square1 : Math  Operator=square  SaturateOnIntegerOverflow=on
  Square2 : Math  Operator=square  SaturateOnIntegerOverflow=on
  Sum : Sum  Inputs=|+++
  Terminator : Terminator
  Terminator1 : Terminator
  P_wind : Outport
  wires:
  Wind Vector/1 -> Demux/1
  Demux/1 -> Square/1
  Demux/2 -> Square1/1
  Demux/3 -> Square2/1
  Square/1 -> Sum/1
  Square1/1 -> Sum/2
  Square2/1 -> Sum/3
  Sum/1 -> Sqrt/1
  Gain/1 -> Multiply/1
  Gain1/1 -> Multiply/2
  Multiply/1 -> P_wind/1
  Math Function/1 -> Gain/1
  Sqrt/1 -> Math Function/1
  Constant/1 -> Math Function/2
  Demux1/1 -> Gain1/1
  Radius/1 -> Demux1/1
  Demux1/3 -> Terminator/1
  Demux1/2 -> Terminator1/1

== system Three_blade_H_VAWT_Model/3bladeHVAWT with Generator/take z1 ==
  In1 : Inport
  Demux : Demux  Outputs=3
  Terminator : Terminator
  Terminator1 : Terminator
  Out1 : Outport
  wires:
  Demux/3 -> Out1/1  "Aero Torque Net"
  Demux/2 -> Terminator1/1
  Demux/1 -> Terminator/1
  In1/1 -> Demux/1

== system Three_blade_H_VAWT_Model/3bladeHVAWT with Generator/take z2 ==
  In1 : Inport
  Demux : Demux  Outputs=3
  Terminator : Terminator
  Terminator1 : Terminator
  Out1 : Outport
  wires:
  In1/1 -> Demux/1
  Demux/1 -> Terminator/1
  Demux/2 -> Terminator1/1
  Demux/3 -> Out1/1  "Aero Torque Net"

== system Three_blade_H_VAWT_Model/3bladeHVAWT with Generator/take z3 ==
  In1 : Inport
  Demux : Demux  Outputs=3
  Terminator : Terminator
  Terminator1 : Terminator
  Out1 : Outport
  wires:
  In1/1 -> Demux/1
  Demux/1 -> Terminator/1
  Demux/2 -> Terminator1/1
  Demux/3 -> Out1/1  "Aero Torque Net"

== system Three_blade_H_VAWT_Model/3bladeHVAWT with Generator/take z4 ==
  In1 : Inport
  Demux : Demux  Outputs=3
  Terminator : Terminator
  Terminator1 : Terminator
  Out1 : Outport
  wires:
  Demux/3 -> Out1/1  "Aero Torque Net"
  Demux/2 -> Terminator1/1
  Demux/1 -> Terminator/1
  In1/1 -> Demux/1

== system Three_blade_H_VAWT_Model/Control/Pitch Control (aoa feedback) Gain Scheduled1 ==
  In1 : Inport
  wind_measure : Inport  Port=2
  Bus Selector : BusSelector  OutputSignals=aoa 1,aoa 2,aoa 3
  Dot Product : DotProduct  InputSameDT=on  OutDataTypeStr=Inherit: Inherit via internal rule
  Multiply : Product
  Multiply1 : Product
  Multiply2 : Product
  Mux : Mux  Inputs=3
  Sqrt : Sqrt  SaturateOnIntegerOverflow=on
  Tunings (20m fixed rad) : Lookup_n-D  NumberOfTableDimensions=1  BreakpointsForDimension1=[0:20]  Table=[0,0,0,0,0,-0.143,-0.28,-0.385,-0.464,-0.527,-0.578,-0.619,0,0,0,0,0,0,0,0,0]  InternalRulePriority=Speed  RndMeth=Simplest  InputSameDT=on
  Pitch Command : Outport
  wires:
  Dot Product/1 -> Sqrt/1
  Sqrt/1 -> Tunings (20m fixed rad)/1
  Tunings (20m fixed rad)/1 -> Multiply/1, Multiply1/1, Multiply2/1
  wind_measure/1 -> Dot Product/2, Dot Product/1
  Mux/1 -> Pitch Command/1
  Multiply2/1 -> Mux/3  "pitch 3"
  Multiply1/1 -> Mux/2  "pitch 2"
  Multiply/1 -> Mux/1  "pitch 1"
  Bus Selector/2 -> Multiply1/2  "<aoa 2>"
  Bus Selector/3 -> Multiply2/2  "<aoa 3>"
  Bus Selector/1 -> Multiply/2  "<aoa 1>"
  In1/1 -> Bus Selector/1

== system Three_blade_H_VAWT_Model/Control/Pitch Control (aoa feedback)1 ==
  In1 : Inport
  Bus Selector : BusSelector  OutputSignals=aoa 1,aoa 2,aoa 3
  Gain : Gain  Gain=-0.3
  Gain1 : Gain  Gain=-0.3
  Gain2 : Gain  Gain=-0.3
  Mux : Mux  Inputs=3
  Pitch Command : Outport
  wires:
  Mux/1 -> Pitch Command/1
  Gain2/1 -> Mux/3  "pitch 3"
  Gain1/1 -> Mux/2  "pitch 2"
  Gain/1 -> Mux/1  "pitch 1"
  Bus Selector/2 -> Gain1/1  "<aoa 2>"
  Bus Selector/3 -> Gain2/1  "<aoa 3>"
  Bus Selector/1 -> Gain/1  "<aoa 1>"
  In1/1 -> Bus Selector/1

== system Three_blade_H_VAWT_Model/Control/Pitch Control (aoa sqrd feedback) ==
  In1 : Inport
  Bus Selector : BusSelector  OutputSignals=aoa 1,aoa 2,aoa 3
  Gain : Gain  Gain=-0.02
  Gain1 : Gain  Gain=-0.02
  Gain3 : Gain  Gain=-0.02
  Math Function : Math  Operator=square  SaturateOnIntegerOverflow=on
  Math Function1 : Math  Operator=square  SaturateOnIntegerOverflow=on
  Math Function2 : Math  Operator=square  SaturateOnIntegerOverflow=on
  Mux : Mux  Inputs=3
  Product : Product
  Product1 : Product
  Product2 : Product
  Sign : Signum
  Sign1 : Signum
  Sign2 : Signum
  Pitch Command : Outport
  wires:
  In1/1 -> Bus Selector/1
  Bus Selector/1 -> Sign/1, Math Function/1  "<aoa 1>"
  Gain/1 -> Mux/1  "pitch 1"
  Gain3/1 -> Mux/2  "pitch 2"
  Gain1/1 -> Mux/3  "pitch 3"
  Mux/1 -> Pitch Command/1
  Math Function/1 -> Product/2
  Sign/1 -> Product/1
  Product/1 -> Gain/1
  Product1/1 -> Gain3/1
  Math Function1/1 -> Product1/2
  Sign1/1 -> Product1/1
  Product2/1 -> Gain1/1
  Math Function2/1 -> Product2/2
  Sign2/1 -> Product2/1
  Bus Selector/3 -> Sign2/1, Math Function2/1  "<aoa 3>"
  Bus Selector/2 -> Sign1/1, Math Function1/1  "<aoa 2>"

== system Three_blade_H_VAWT_Model/3bladeHVAWT with Generator/Blade Aerodymanics/Finite Wing Correction ==
  Cl' : Inport
  Cd' : Inport  Port=2
  Constant1 : Constant  Value=AR
  Terminator : Terminator
  Cl : Outport
  Cd : Outport  Port=2
  wires:
  Constant1/1 -> Terminator/1  "AR"
  Cl'/1 -> Cl/1
  Cd'/1 -> Cd/1

== system Three_blade_H_VAWT_Model/3bladeHVAWT with Generator/Blade Aerodymanics/Finite Wing Correction1 ==
  Cl' : Inport
  Cd' : Inport  Port=2
  Constant1 : Constant  Value=AR
  Terminator : Terminator
  Cl : Outport
  Cd : Outport  Port=2
  wires:
  Cd'/1 -> Cd/1
  Cl'/1 -> Cl/1
  Constant1/1 -> Terminator/1  "AR"

== system Three_blade_H_VAWT_Model/3bladeHVAWT with Generator/Blade Aerodymanics/Finite Wing Correction2 ==
  Cl' : Inport
  Cd' : Inport  Port=2
  Constant1 : Constant  Value=AR
  Terminator : Terminator
  Cl : Outport
  Cd : Outport  Port=2
  wires:
  Constant1/1 -> Terminator/1  "AR"
  Cl'/1 -> Cl/1
  Cd'/1 -> Cd/1

== system Three_blade_H_VAWT_Model/3bladeHVAWT with Generator/Blade Aerodymanics/Lift Align1 ==
  AoA : Inport
  L_mag : Inport  Port=2
  Blade_Pos : Inport  Port=3
  Constant : Constant  Value=0
  Demux : Demux  Outputs=3
  Demux1 : Demux  Outputs=2
  Gain : Gain  Gain=pi/180
  MATLAB Function : MATLAB Function  TreatAsAtomicUnit=on
  Mux : Mux  Inputs=2
  Mux1 : Mux  Inputs=3
  Normalization : dspmathops/Normalization  NormType=2-norm  Bias=1e-10  NormOver=Each column  Dimension=1  roundingMode=Floor  overflowMode=off  accumDataTypeStr=Inherit: Same as product output  accumLastDataTypeStr=Inherit: Same as product output  outputDataTypeStr=Inherit: Same as product output  outputMin=[]  outputMax=[]  outputLastDataTypeStr=Inherit: Same as product output
      settings: SourceProductName=DSP System Toolbox
  Product : Product
  Product1 : Product  Multiplication=Matrix(*)
  Terminator : Terminator
  Lift_Vec : Outport
  wires:
  Constant/1 -> Mux1/3
  Mux1/1 -> Lift_Vec/1
  Demux1/2 -> Mux1/2
  Demux1/1 -> Mux1/1
  Mux/1 -> Product1/2
  Demux/3 -> Terminator/1
  Demux/2 -> Mux/2
  Demux/1 -> Mux/1
  Product/1 -> Demux/1
  Blade_Pos/1 -> Normalization/1
  Normalization/1 -> Product/2
  L_mag/1 -> Product/1
  AoA/1 -> Gain/1
  Gain/1 -> MATLAB Function/1(Theta)
  Product1/1 -> Demux1/1
  MATLAB Function/1(Mat) -> Product1/1

== system Three_blade_H_VAWT_Model/3bladeHVAWT with Generator/Blade Aerodymanics/Lift Align2 ==
  AoA : Inport
  L_mag : Inport  Port=2
  Blade_Pos : Inport  Port=3
  Constant : Constant  Value=0
  Demux : Demux  Outputs=3
  Demux1 : Demux  Outputs=2
  Gain : Gain  Gain=pi/180
  MATLAB Function : MATLAB Function  TreatAsAtomicUnit=on
  Mux : Mux  Inputs=2
  Mux1 : Mux  Inputs=3
  Normalization : dspmathops/Normalization  NormType=2-norm  Bias=1e-10  NormOver=Each column  Dimension=1  roundingMode=Floor  overflowMode=off  accumDataTypeStr=Inherit: Same as product output  accumLastDataTypeStr=Inherit: Same as product output  outputDataTypeStr=Inherit: Same as product output  outputMin=[]  outputMax=[]  outputLastDataTypeStr=Inherit: Same as product output
      settings: SourceProductName=DSP System Toolbox
  Product : Product
  Product1 : Product  Multiplication=Matrix(*)
  Terminator : Terminator
  Lift_Vec : Outport
  wires:
  MATLAB Function/1(Mat) -> Product1/1
  Product1/1 -> Demux1/1
  Gain/1 -> MATLAB Function/1(Theta)
  AoA/1 -> Gain/1
  L_mag/1 -> Product/1
  Normalization/1 -> Product/2
  Blade_Pos/1 -> Normalization/1
  Product/1 -> Demux/1
  Demux/1 -> Mux/1
  Demux/2 -> Mux/2
  Demux/3 -> Terminator/1
  Mux/1 -> Product1/2
  Demux1/1 -> Mux1/1
  Demux1/2 -> Mux1/2
  Mux1/1 -> Lift_Vec/1
  Constant/1 -> Mux1/3

== system Three_blade_H_VAWT_Model/3bladeHVAWT with Generator/Blade Aerodymanics/Lift Align3 ==
  AoA : Inport
  L_mag : Inport  Port=2
  Blade_Pos : Inport  Port=3
  Constant : Constant  Value=0
  Demux : Demux  Outputs=3
  Demux1 : Demux  Outputs=2
  Gain : Gain  Gain=pi/180
  MATLAB Function : MATLAB Function  TreatAsAtomicUnit=on
  Mux : Mux  Inputs=2
  Mux1 : Mux  Inputs=3
  Normalization : dspmathops/Normalization  NormType=2-norm  Bias=1e-10  NormOver=Each column  Dimension=1  roundingMode=Floor  overflowMode=off  accumDataTypeStr=Inherit: Same as product output  accumLastDataTypeStr=Inherit: Same as product output  outputDataTypeStr=Inherit: Same as product output  outputMin=[]  outputMax=[]  outputLastDataTypeStr=Inherit: Same as product output
      settings: SourceProductName=DSP System Toolbox
  Product : Product
  Product1 : Product  Multiplication=Matrix(*)
  Terminator : Terminator
  Lift_Vec : Outport
  wires:
  MATLAB Function/1(Mat) -> Product1/1
  Product1/1 -> Demux1/1
  Gain/1 -> MATLAB Function/1(Theta)
  AoA/1 -> Gain/1
  L_mag/1 -> Product/1
  Normalization/1 -> Product/2
  Blade_Pos/1 -> Normalization/1
  Product/1 -> Demux/1
  Demux/1 -> Mux/1
  Demux/2 -> Mux/2
  Demux/3 -> Terminator/1
  Mux/1 -> Product1/2
  Demux1/1 -> Mux1/1
  Demux1/2 -> Mux1/2
  Mux1/1 -> Lift_Vec/1
  Constant/1 -> Mux1/3

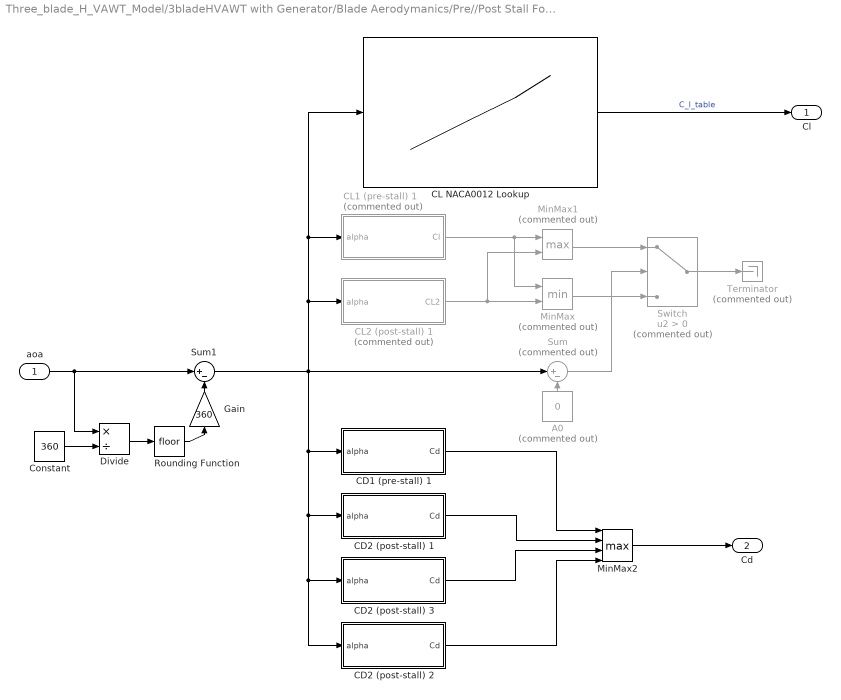
== system Three_blade_H_VAWT_Model/3bladeHVAWT with Generator/Blade Aerodymanics/Pre//Post Stall Foil Model NACA 0012 ==
  aoa : Inport
  A0 : Constant  Commented=on  Value=0
  CD1 (pre-stall) 1 : Subsystem
  CD2 (post-stall) 1 : Subsystem
  CD2 (post-stall) 2 : Subsystem
  CD2 (post-stall) 3 : Subsystem
  CL NACA0012 Lookup : Lookup_n-D  NumberOfTableDimensions=1  BreakpointsForDimension1=[0:1:360]  Table=C_l_NACA0012_spline  InternalRulePriority=Speed  RndMeth=Simplest  InputSameDT=on
  CL1 (pre-stall) 1 : Subsystem  Commented=on
  CL2 (post-stall) 1 : Subsystem  Commented=on
  Constant : Constant  Value=360
  Divide : Product  Inputs=*/
  Gain : Gain  Gain=360
  MinMax : MinMax  Commented=on  Inputs=2
  MinMax1 : MinMax  Commented=on  Function=max  Inputs=2
  MinMax2 : MinMax  Function=max  Inputs=4
  Rounding Function : Rounding
  Sum : Sum  Commented=on  Inputs=|+-
  Sum1 : Sum  Inputs=|+-
  Switch : Switch  Commented=on  Criteria=u2 > Threshold
  Terminator : Terminator  Commented=on
  Cl : Outport
  Cd : Outport  Port=2
  wires:
  Sum/1 -> Switch/2
  MinMax2/1 -> Cd/1
  Switch/1 -> Terminator/1
  A0/1 -> Sum/2
  CD2 (post-stall) 1/1(Cd) -> MinMax2/2
  CD1 (pre-stall) 1/1(Cd) -> MinMax2/1
  MinMax1/1 -> Switch/1
  CL1 (pre-stall) 1/1(Cl) -> MinMax1/1, MinMax/1
  CL2 (post-stall) 1/1(CL2) -> MinMax1/2, MinMax/2
  MinMax/1 -> Switch/3
  aoa/1 -> Divide/1, Sum1/1
  Constant/1 -> Divide/2
  Divide/1 -> Rounding Function/1
  Rounding Function/1 -> Gain/1
  Sum1/1 -> CD2 (post-stall) 3/1(alpha), CD2 (post-stall) 2/1(alpha), CD2 (post-stall) 1/1(alpha), CD1 (pre-stall) 1/1(alpha), CL NACA0012 Lookup/1, CL1 (pre-stall) 1/1(alpha), CL2 (post-stall) 1/1(alpha), Sum/1
  CL NACA0012 Lookup/1 -> Cl/1  "C_l_table"
  Gain/1 -> Sum1/2
  CD2 (post-stall) 2/1(Cd) -> MinMax2/4
  CD2 (post-stall) 3/1(Cd) -> MinMax2/3

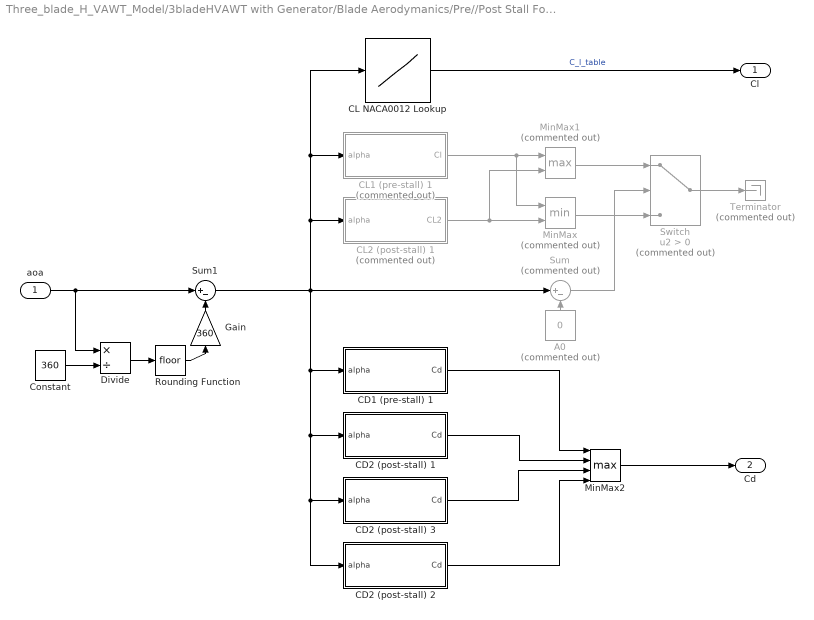
== system Three_blade_H_VAWT_Model/3bladeHVAWT with Generator/Blade Aerodymanics/Pre//Post Stall Foil Model NACA 0012 (2) ==
  aoa : Inport
  A0 : Constant  Commented=on  Value=0
  CD1 (pre-stall) 1 : Subsystem
  CD2 (post-stall) 1 : Subsystem
  CD2 (post-stall) 2 : Subsystem
  CD2 (post-stall) 3 : Subsystem
  CL NACA0012 Lookup : Lookup_n-D  NumberOfTableDimensions=1  BreakpointsForDimension1=[0:1:360]  Table=C_l_NACA0012_spline  InternalRulePriority=Speed  RndMeth=Simplest  InputSameDT=on
  CL1 (pre-stall) 1 : Subsystem  Commented=on
  CL2 (post-stall) 1 : Subsystem  Commented=on
  Constant : Constant  Value=360
  Divide : Product  Inputs=*/
  Gain : Gain  Gain=360
  MinMax : MinMax  Commented=on  Inputs=2
  MinMax1 : MinMax  Commented=on  Function=max  Inputs=2
  MinMax2 : MinMax  Function=max  Inputs=4
  Rounding Function : Rounding
  Sum : Sum  Commented=on  Inputs=|+-
  Sum1 : Sum  Inputs=|+-
  Switch : Switch  Commented=on  Criteria=u2 > Threshold
  Terminator : Terminator  Commented=on
  Cl : Outport
  Cd : Outport  Port=2
  wires:
  CD2 (post-stall) 3/1(Cd) -> MinMax2/3
  CD2 (post-stall) 2/1(Cd) -> MinMax2/4
  Gain/1 -> Sum1/2
  CL NACA0012 Lookup/1 -> Cl/1  "C_l_table"
  Sum1/1 -> Sum/1, CL2 (post-stall) 1/1(alpha), CL1 (pre-stall) 1/1(alpha), CL NACA0012 Lookup/1, CD1 (pre-stall) 1/1(alpha), CD2 (post-stall) 1/1(alpha), CD2 (post-stall) 2/1(alpha), CD2 (post-stall) 3/1(alpha)
  Rounding Function/1 -> Gain/1
  Divide/1 -> Rounding Function/1
  Constant/1 -> Divide/2
  aoa/1 -> Sum1/1, Divide/1
  MinMax/1 -> Switch/3
  CL2 (post-stall) 1/1(CL2) -> MinMax/2, MinMax1/2
  CL1 (pre-stall) 1/1(Cl) -> MinMax/1, MinMax1/1
  MinMax1/1 -> Switch/1
  CD1 (pre-stall) 1/1(Cd) -> MinMax2/1
  CD2 (post-stall) 1/1(Cd) -> MinMax2/2
  A0/1 -> Sum/2
  Switch/1 -> Terminator/1
  MinMax2/1 -> Cd/1
  Sum/1 -> Switch/2

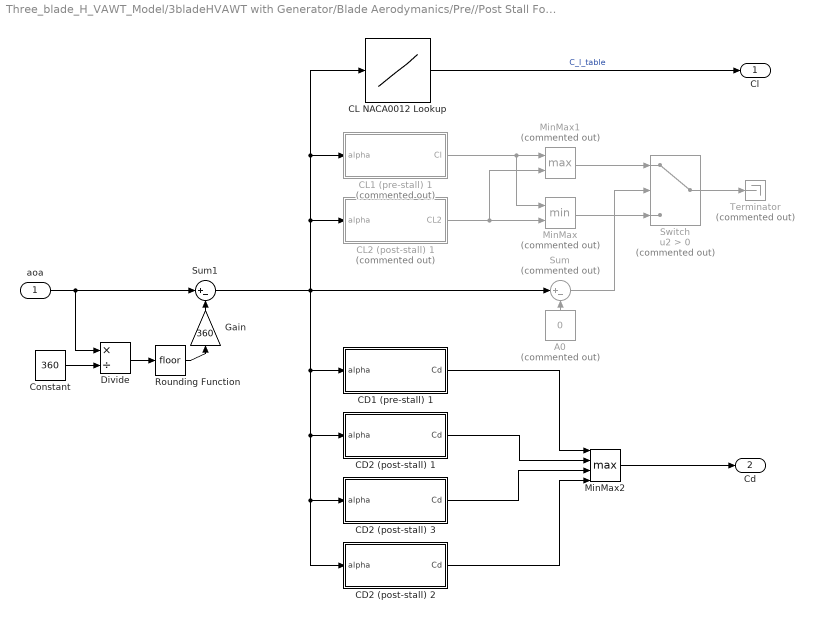
== system Three_blade_H_VAWT_Model/3bladeHVAWT with Generator/Blade Aerodymanics/Pre//Post Stall Foil Model NACA 0012 (3) ==
  aoa : Inport
  A0 : Constant  Commented=on  Value=0
  CD1 (pre-stall) 1 : Subsystem
  CD2 (post-stall) 1 : Subsystem
  CD2 (post-stall) 2 : Subsystem
  CD2 (post-stall) 3 : Subsystem
  CL NACA0012 Lookup : Lookup_n-D  NumberOfTableDimensions=1  BreakpointsForDimension1=[0:1:360]  Table=C_l_NACA0012_spline  InternalRulePriority=Speed  RndMeth=Simplest  InputSameDT=on
  CL1 (pre-stall) 1 : Subsystem  Commented=on
  CL2 (post-stall) 1 : Subsystem  Commented=on
  Constant : Constant  Value=360
  Divide : Product  Inputs=*/
  Gain : Gain  Gain=360
  MinMax : MinMax  Commented=on  Inputs=2
  MinMax1 : MinMax  Commented=on  Function=max  Inputs=2
  MinMax2 : MinMax  Function=max  Inputs=4
  Rounding Function : Rounding
  Sum : Sum  Commented=on  Inputs=|+-
  Sum1 : Sum  Inputs=|+-
  Switch : Switch  Commented=on  Criteria=u2 > Threshold
  Terminator : Terminator  Commented=on
  Cl : Outport
  Cd : Outport  Port=2
  wires:
  Sum/1 -> Switch/2
  MinMax2/1 -> Cd/1
  Switch/1 -> Terminator/1
  A0/1 -> Sum/2
  CD2 (post-stall) 1/1(Cd) -> MinMax2/2
  CD1 (pre-stall) 1/1(Cd) -> MinMax2/1
  MinMax1/1 -> Switch/1
  CL1 (pre-stall) 1/1(Cl) -> MinMax1/1, MinMax/1
  CL2 (post-stall) 1/1(CL2) -> MinMax1/2, MinMax/2
  MinMax/1 -> Switch/3
  aoa/1 -> Divide/1, Sum1/1
  Constant/1 -> Divide/2
  Divide/1 -> Rounding Function/1
  Rounding Function/1 -> Gain/1
  Sum1/1 -> CD2 (post-stall) 3/1(alpha), CD2 (post-stall) 2/1(alpha), CD2 (post-stall) 1/1(alpha), CD1 (pre-stall) 1/1(alpha), CL NACA0012 Lookup/1, CL1 (pre-stall) 1/1(alpha), CL2 (post-stall) 1/1(alpha), Sum/1
  CL NACA0012 Lookup/1 -> Cl/1  "C_l_table"
  Gain/1 -> Sum1/2
  CD2 (post-stall) 2/1(Cd) -> MinMax2/4
  CD2 (post-stall) 3/1(Cd) -> MinMax2/3

== system Three_blade_H_VAWT_Model/3bladeHVAWT with Generator/Blade Geometry Mk2/Vector 2 norm ==
  In1 : Inport
  Dot Product : DotProduct  InputSameDT=on  OutDataTypeStr=Inherit: Inherit via internal rule
  Sqrt : Sqrt  SaturateOnIntegerOverflow=on
  Out1 : Outport
  wires:
  In1/1 -> Dot Product/2, Dot Product/1
  Dot Product/1 -> Sqrt/1
  Sqrt/1 -> Out1/1

== system Three_blade_H_VAWT_Model/3bladeHVAWT with Generator/Blade Geometry Mk2/Vector 2 norm1 ==
  In1 : Inport
  Dot Product : DotProduct  InputSameDT=on  OutDataTypeStr=Inherit: Inherit via internal rule
  Sqrt : Sqrt  SaturateOnIntegerOverflow=on
  Out1 : Outport
  wires:
  Sqrt/1 -> Out1/1
  Dot Product/1 -> Sqrt/1
  In1/1 -> Dot Product/1, Dot Product/2

== system Three_blade_H_VAWT_Model/3bladeHVAWT with Generator/Blade Geometry Mk2/Vector 2 norm2 ==
  In1 : Inport
  Dot Product : DotProduct  InputSameDT=on  OutDataTypeStr=Inherit: Inherit via internal rule
  Sqrt : Sqrt  SaturateOnIntegerOverflow=on
  Out1 : Outport
  wires:
  In1/1 -> Dot Product/2, Dot Product/1
  Dot Product/1 -> Sqrt/1
  Sqrt/1 -> Out1/1

== system Three_blade_H_VAWT_Model/3bladeHVAWT with Generator/Blade Geometry Mk2/Vector 2 norm3 ==
  In1 : Inport
  Dot Product : DotProduct  InputSameDT=on  OutDataTypeStr=Inherit: Inherit via internal rule
  Sqrt : Sqrt  SaturateOnIntegerOverflow=on
  Out1 : Outport
  wires:
  Sqrt/1 -> Out1/1
  Dot Product/1 -> Sqrt/1
  In1/1 -> Dot Product/1, Dot Product/2

== system Three_blade_H_VAWT_Model/3bladeHVAWT with Generator/Blade Geometry Mk2/Vector 2 norm4 ==
  In1 : Inport
  Dot Product : DotProduct  InputSameDT=on  OutDataTypeStr=Inherit: Inherit via internal rule
  Sqrt : Sqrt  SaturateOnIntegerOverflow=on
  Out1 : Outport
  wires:
  In1/1 -> Dot Product/2, Dot Product/1
  Dot Product/1 -> Sqrt/1
  Sqrt/1 -> Out1/1

== system Three_blade_H_VAWT_Model/3bladeHVAWT with Generator/Blade Geometry Mk2/Vector 2 norm5 ==
  In1 : Inport
  Dot Product : DotProduct  InputSameDT=on  OutDataTypeStr=Inherit: Inherit via internal rule
  Sqrt : Sqrt  SaturateOnIntegerOverflow=on
  Out1 : Outport
  wires:
  Sqrt/1 -> Out1/1
  Dot Product/1 -> Sqrt/1
  In1/1 -> Dot Product/1, Dot Product/2

== system Three_blade_H_VAWT_Model/3bladeHVAWT with Generator/Blade Aerodymanics/Pre//Post Stall Foil Model NACA 0012/CD1 (pre-stall) 1 ==
  alpha : Inport
  A0 : Constant  Value=A0
  ACD1 : Constant  Value=ACD1
  CD0 : Constant  Value=CD0
  CD1_max : Constant  Value=CD1_max
  Constant1 : Constant  Value=ACD1
  Divide : Product  Inputs=*/
  MATLAB Function : MATLAB Function  TreatAsAtomicUnit=on
  MATLAB Function1 : MATLAB Function  TreatAsAtomicUnit=on
  Math Function : Math  Operator=square  SaturateOnIntegerOverflow=on
  Product : Product
  Product1 : Product
  Scope : Scope
  Scope1 : Scope
  Scope2 : Scope
  Sum : Sum  Inputs=|++
  Sum1 : Sum  Inputs=-+|
  Sum2 : Sum  Inputs=|-+
  Sum3 : Sum  Inputs=|+-
  Cd : Outport
  wires:
  alpha/1 -> MATLAB Function/1(alpha), Scope1/1, MATLAB Function1/1("alpha ")
  CD0/1 -> Sum1/1, Sum/1
  CD1_max/1 -> Sum1/2
  Sum1/1 -> Product/1
  A0/1 -> Sum3/2, Sum2/1
  ACD1/1 -> Sum3/1
  Sum2/1 -> Divide/1
  Sum3/1 -> Divide/2
  Divide/1 -> Math Function/1
  Math Function/1 -> Product/2
  Product/1 -> Sum/2
  Sum/1 -> Product1/1
  Product1/1 -> Cd/1
  Constant1/1 -> MATLAB Function/2(ACD1)
  MATLAB Function/1(y) -> Product1/2, Scope/1
  MATLAB Function1/1(alpha) -> Scope2/1, Sum2/2
